simulink model "helicopter_robust_model"  (R2023b)
settings: Solver=VariableStepAuto  StartTime=0.0  StopTime=20  MaxStep=0.01  RelTol=1e-5
libraries: cstblocks x8
settings Model: Creator=torb  LastModifiedBy=torb
settings OptimizationCC: DefaultParameterBehavior=Inlined  BufferReuse=off
settings DebuggingCC: InitInArrayFormatMsg=none

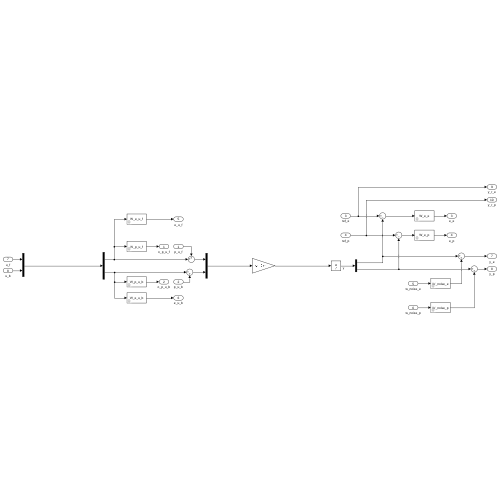
[thumbnail: Simulink's stored preview of the top-level diagram]
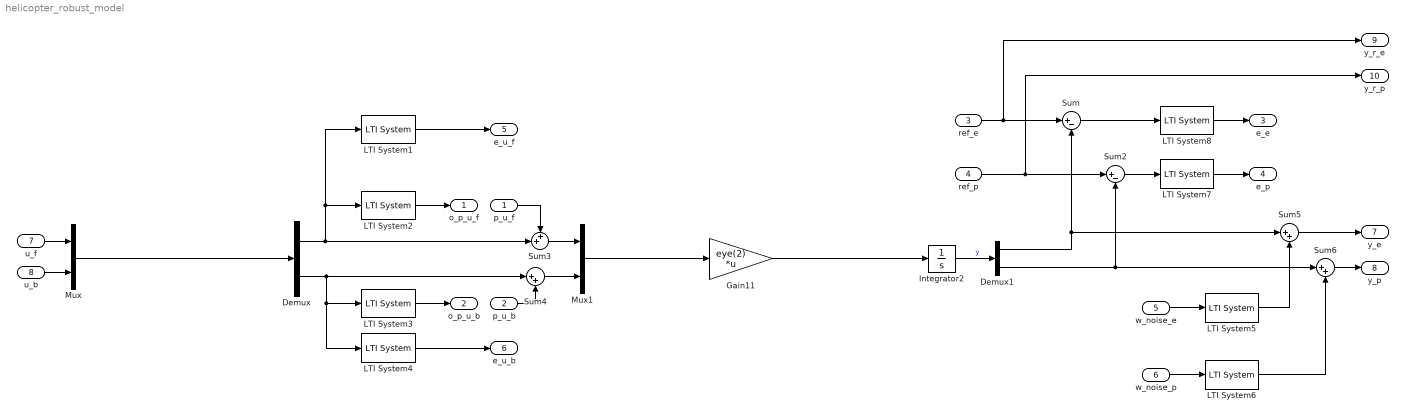
== system helicopter_robust_model ==
  p_u_f : Inport
  p_u_b : Inport  Port=2
  ref_e : Inport  Port=3
  ref_p : Inport  Port=4
  w_noise_e : Inport  Port=5
  w_noise_p : Inport  Port=6
  u_f : Inport  Port=7
  u_b : Inport  Port=8
  Demux : Demux  Outputs=2
  Demux1 : Demux  Outputs=2
  Gain11 : Gain  Gain=eye(2)  Multiplication=Matrix(K*u)
  Integrator2 : Integrator
  LTI System1 : cstblocks/LTI System  sys=W_e_u_f  IC=[]  PadeOrder=0
  LTI System2 : cstblocks/LTI System  sys=W_p_u_f  IC=[]  PadeOrder=0
  LTI System3 : cstblocks/LTI System  sys=W_p_u_b  IC=[]  PadeOrder=0
  LTI System4 : cstblocks/LTI System  sys=W_e_u_b  IC=[]  PadeOrder=0
  LTI System5 : cstblocks/LTI System  sys=W_noise_e  IC=[]  PadeOrder=0
  LTI System6 : cstblocks/LTI System  sys=W_noise_p  IC=[]  PadeOrder=0
  LTI System7 : cstblocks/LTI System  sys=W_e_p  IC=[]  PadeOrder=0
  LTI System8 : cstblocks/LTI System  sys=W_e_e  IC=[]  PadeOrder=0
  Mux : Mux  Inputs=2
  Mux1 : Mux  Inputs=2
  Sum : Sum  Inputs=|+-
  Sum2 : Sum  Inputs=|+-
  Sum3 : Sum  Inputs=++|
  Sum4 : Sum  Inputs=|++
  Sum5 : Sum  Inputs=|++
  Sum6 : Sum  Inputs=|++
  o_p_u_f : Outport
  o_p_u_b : Outport  Port=2
  e_e : Outport  Port=3
  e_p : Outport  Port=4
  e_u_f : Outport  Port=5
  e_u_b : Outport  Port=6
  y_e : Outport  Port=7
  y_p : Outport  Port=8
  y_r_e : Outport  Port=9
  y_r_p : Outport  Port=10
  wires:
  Integrator2/1 -> Demux1/1  "y"
  u_b/1 -> Mux/2
  u_f/1 -> Mux/1
  ref_e/1 -> Sum/1, y_r_e/1
  ref_p/1 -> Sum2/1, y_r_p/1
  Demux1/1 -> Sum/2, Sum5/1
  Demux1/2 -> Sum6/1, Sum2/2
  LTI System2/1 -> o_p_u_f/1
  Demux/1 -> LTI System2/1, LTI System1/1, Sum3/2
  p_u_f/1 -> Sum3/1
  Sum3/1 -> Mux1/1
  Sum4/1 -> Mux1/2
  Demux/2 -> Sum4/1, LTI System4/1, LTI System3/1
  p_u_b/1 -> Sum4/2
  LTI System3/1 -> o_p_u_b/1
  w_noise_e/1 -> LTI System5/1
  w_noise_p/1 -> LTI System6/1
  Sum5/1 -> y_e/1
  Sum6/1 -> y_p/1
  LTI System6/1 -> Sum6/2
  LTI System5/1 -> Sum5/2
  LTI System1/1 -> e_u_f/1
  LTI System4/1 -> e_u_b/1
  LTI System8/1 -> e_e/1
  Sum2/1 -> LTI System7/1
  LTI System7/1 -> e_p/1
  Mux/1 -> Demux/1
  Mux1/1 -> Gain11/1
  Gain11/1 -> Integrator2/1
  Sum/1 -> LTI System8/1
